simulink model "w2p3"  (R2020a)
settings: Solver=VariableStepAuto  StartTime=0.0  StopTime=120  RelTol=1e-3
values from neighbouring files (symbols this model uses):
  b = 50    [w2p3.mat]
  m = 1000    [w2p3.mat]
settings Model: Creator=Shubham  LastModifiedBy=Shubham

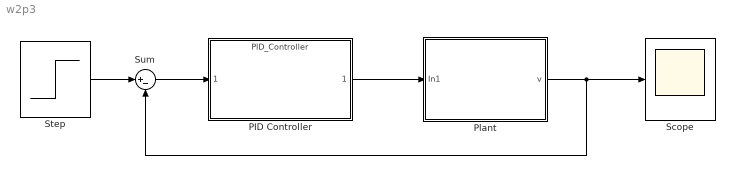
== system w2p3 ==
  PID Controller : ModelReference  ModelNameDialog=PID_Controller  SimulationMode=Normal  ModelReferenceVersion=1.4
  Plant : Subsystem
  Scope : Scope
  Step : Step  Time=0  After=u  SampleTime=0
  Sum : Sum  Inputs=|+-
  wires:
  Step/1 -> Sum/1
  Sum/1 -> PID Controller/1
  PID Controller/1 -> Plant/1(In1)
  Plant/1(v) -> Sum/2, Scope/1

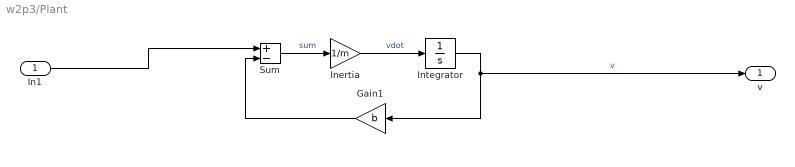
== system w2p3/Plant ==
  In1 : Inport
  Gain1 : Gain  Gain=b
  Inertia : Gain  Gain=1/m
  Integrator : Integrator
  Sum : Sum  Inputs=+-
  v : Outport
  wires:
  Gain1/1 -> Sum/2
  In1/1 -> Sum/1
  Integrator/1 -> v/1, Gain1/1  "v"
  Inertia/1 -> Integrator/1  "vdot"
  Sum/1 -> Inertia/1  "sum"
